simulink model "generacioAudio"  (R2020b)
settings: Solver=VariableStepAuto  StartTime=0.0  StopTime=37  RelTol=1e-3
libraries: commdigbbndpm3 x1, dspvision x1, commutil2 x1
settings Model: Creator=dlap-  LastModifiedBy=dlap-

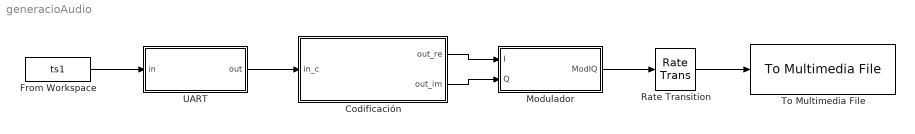
== system generacioAudio ==
  Codificación : Subsystem
  From Workspace : FromWorkspace  VariableName=ts1  SampleTime=1  Interpolate=off  OutputAfterFinalValue=Setting to zero
  Modulador : Subsystem
  Rate Transition : RateTransition  OutPortSampleTime=1/44100
  To Multimedia File : dspvision/To Multimedia File  outputFilename=D:\dlap-\Documents\Diana UNAM\Sistemas de Comunicaciones\ProyectoFinal\audiogout.wav  streamSelection=Audio only  videoCompressor=None (uncompressed)  audioCompressor=None (uncompressed)  imagePorts=Separate color signals  fileType=WAV  audioDatatype=16-bit integer  fourcc=RGB  videoQuality=75  mj2000CompFactor=10
  UART : Subsystem
  wires:
  From Workspace/1 -> UART/1(in)
  UART/1(out) -> Codificación/1(in_c)
  Codificación/1(out_re) -> Modulador/1(I)
  Codificación/2(out_im) -> Modulador/2(Q)
  Modulador/1(ModIQ) -> Rate Transition/1
  Rate Transition/1 -> To Multimedia File/1

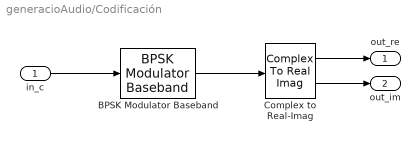
== system generacioAudio/Codificación ==
  in_c : Inport
  BPSK Modulator Baseband : commdigbbndpm3/BPSK Modulator Baseband  Ph=0  outDtype=double  outWordLen=16  outUDDataType=sfix(16)  outFracLenMode=Best precision  outFracLen=15  outDataTypeStr=double  outLastDataTypeStr=double
  Complex to Real-Imag : ComplexToRealImag
  out_re : Outport
  out_im : Outport  Port=2
  wires:
  BPSK Modulator Baseband/1 -> Complex to Real-Imag/1
  in_c/1 -> BPSK Modulator Baseband/1
  Complex to Real-Imag/1 -> out_re/1
  Complex to Real-Imag/2 -> out_im/1

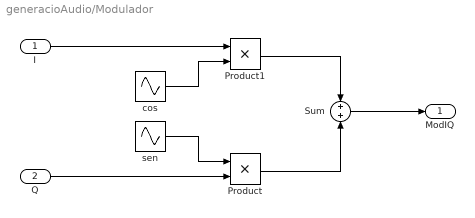
== system generacioAudio/Modulador ==
  I : Inport
  Q : Inport  Port=2
  Product : Product
  Product1 : Product
  Sum : Sum  Inputs=+|+
  cos : Sin  Frequency=2*pi*4000  Phase=pi/2  SampleTime=0
  sen : Sin  Frequency=2*pi*4000  SampleTime=0
  ModIQ : Outport
  wires:
  Product/1 -> Sum/2
  Product1/1 -> Sum/1
  cos/1 -> Product1/2
  sen/1 -> Product/1
  Q/1 -> Product/2
  Sum/1 -> ModIQ/1
  I/1 -> Product1/1

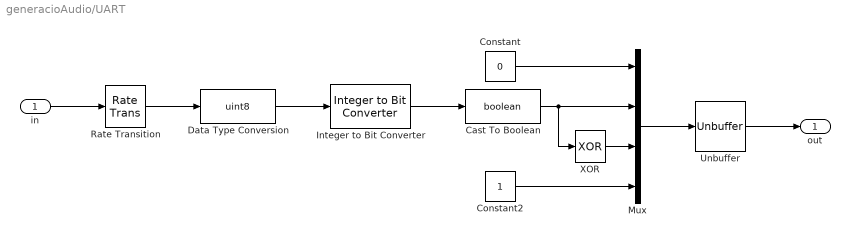
== system generacioAudio/UART ==
  in : Inport
  Cast To Boolean : DataTypeConversion  OutDataTypeStr=boolean
  Constant : Constant  Value=0  OutDataTypeStr=boolean
  Constant2 : Constant  OutDataTypeStr=boolean
  Data Type Conversion : DataTypeConversion  OutDataTypeStr=uint8
  Integer to Bit Converter : commutil2/Integer to Bit Converter  nbits=8  signedInputValues=Unsigned  bitOrder=MSB first  outDtype=uint8
  Mux : Mux
  Rate Transition : RateTransition  OutPortSampleTime=1/44100
  Unbuffer : Unbuffer
  XOR : Logic  Operator=XOR  Inputs=1  IconShape=distinctive  AllPortsSameDT=off  OutDataTypeStr=boolean
  out : Outport
  wires:
  Cast To Boolean/1 -> Mux/2, XOR/1
  Integer to Bit Converter/1 -> Cast To Boolean/1
  Constant2/1 -> Mux/4
  Constant/1 -> Mux/1
  Rate Transition/1 -> Data Type Conversion/1
  Data Type Conversion/1 -> Integer to Bit Converter/1
  Mux/1 -> Unbuffer/1
  XOR/1 -> Mux/3
  Unbuffer/1 -> out/1
  in/1 -> Rate Transition/1
